simulink model "jacobian_inverse"  (R2020a)
settings: Solver=VariableStepAuto  StartTime=0.0  StopTime=1  RelTol=1e-3
values from neighbouring files (symbols this model uses):
  K = 100*diag([1 1 1])    [JoinScript.m]    (also in alldata.mat = [20.1 11.1 12 0 0 0 11.1 20.1 12 0 0 0 ... (36 elements, 6x6; aux_y2.m = Abb.fkine(q))
  qf = [pi/2 pi/3 pi/12 pi/2 0 pi/2]    [JoinScript.m]    (also in alldata.mat = [1.57079632679 1.0471975512 0.261799387799 1.57079632679 0 1; model_script.m = [pi/6 0 pi/3 pi/4 0 0])
settings Model: Creator=doble  LastModifiedBy=doble

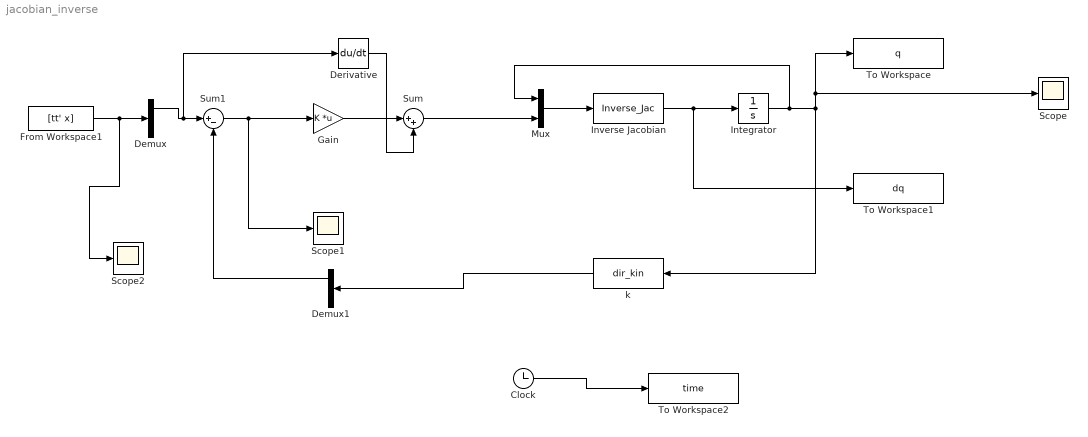
== system jacobian_inverse ==
  Clock : Clock
  Demux : Demux  Outputs=[3 3]
  Demux1 : Demux  Outputs=[3 3]
  Derivative : Derivative
  From Workspace1 : FromWorkspace  VariableName=[tt' x]
  Gain : Gain  Gain=K  Multiplication=Matrix(K*u)
  Integrator : Integrator  InitialCondition=qf
  Inverse Jacobian : MATLABFcn  MATLABFcn=Inverse_Jac  OutputDimensions=6*1
  Mux : Mux  Inputs=[6 3]
  Scope : Scope
  Scope1 : Scope
  Scope2 : Scope
  Sum : Sum  Inputs=|++
  Sum1 : Sum  Inputs=|+-
  To Workspace : ToWorkspace  VariableName=q  SaveFormat=Timeseries  SampleTime=-1
  To Workspace1 : ToWorkspace  VariableName=dq  SaveFormat=Timeseries  SampleTime=-1
  To Workspace2 : ToWorkspace  VariableName=time  SaveFormat=Timeseries  SampleTime=-1
  k : MATLABFcn  MATLABFcn=dir_kin
  wires:
  Integrator/1 -> Mux/1, Scope/1, To Workspace/1, k/1
  Mux/1 -> Inverse Jacobian/1
  Inverse Jacobian/1 -> To Workspace1/1, Integrator/1
  Sum/1 -> Mux/2
  Gain/1 -> Sum/1
  From Workspace1/1 -> Scope2/1, Demux/1
  Sum1/1 -> Scope1/1, Gain/1
  Clock/1 -> To Workspace2/1
  Demux/1 -> Derivative/1, Sum1/1
  k/1 -> Demux1/1
  Demux1/1 -> Sum1/2
  Derivative/1 -> Sum/2
